simulink model "Lab1_open"  (R2024b)
settings: Solver=ode1  StartTime=0.0  StopTime=5  FixedStep=0.002  RelTol=1e-3  EnableMultiTasking=on
undefined symbols (not defined in the file or in its folder): HIL
libraries: quarc_library x3
settings Model: ExtModeTrigDuration=50001  Creator=Mounir  LastModifiedBy=dodso
settings SolverCC: AlgebraicLoopSolver=TrustRegion  PositivePriorityOrder=on
settings DataIOCC: LimitDataPoints=on  SaveFormat=Array  SaveOutput=off  SaveTime=off  ReturnWorkspaceOutputs=off
settings OptimizationCC: LifeSpan=inf
settings DebuggingCC: SolverPrmCheckMsg=warning  UnconnectedInputMsg=warning  UnconnectedOutputMsg=warning  UnconnectedLineMsg=warning  AllowSymbolicDim=off  SFUnexpectedBacktrackingDiag=warning  SFNoUnconditionalDefaultTransitionDiag=warning  SFExecutionAtInitializationDiag=none  ArithmeticOperatorsInVariantConditions=warning
settings HardwareCC: ProdBitPerPointer=32  ProdBitPerSizeT=32  ProdBitPerPtrDiffT=32  ProdLargestAtomicFloat=None  ProdIntDivRoundTo=Undefined  ProdEndianess=Unspecified  ProdWordSize=32  ProdHWDeviceType=32-bit Generic
settings ModelReferenceCC: EnableRefExpFcnMdlSchedulingChecks=on  PropagateSignalLabelsOutOfModel=off
settings SFSimCC: SimUseLocalCustomCode=off  CustomCodeUndefinedFunction=UseInterfaceOnly
settings RTWCC: Description=QUARC Win64 Target  SystemTargetFile=quarc_win64.tlc  TemplateMakefile=quarc_default_tmf  RTWUseLocalCustomCode=off  GPUComputeCapability=3.5
settings CodeAppCC: StateflowObjectComments=on
settings STFCustomTargetCC: TargetPreCompLibLocation=C:\PROGRA~3\QUARC\lib\2015b\win64\release  ConcurrentExecutionCompliant=on  CombineOutputUpdateFcns=on  SystemTargetFile=quarc_win64.tlc
settings GRTTargetCC: TargetPreCompLibLocation=C:\PROGRA~3\QUARC\lib\2015b\win64\release  TargetLangStandard=C89/C90 (ANSI)  ParMdlRefBuildCompliant=off  CompOptLevelCompliant=off  MatFileLogging=off  CPPClassGenCompliant=off  UseToolchainInfoCompliant=off  ExtMode=on  ExtModeMexFile=quarc_comm
settings ConfigComp: CovMetricSettings=dw  CovSaveCumulativeToWorkspaceVar=on  CovSaveSingleToWorkspaceVar=on  CovExternalEMLEnable=off  CovSFcnEnable=off

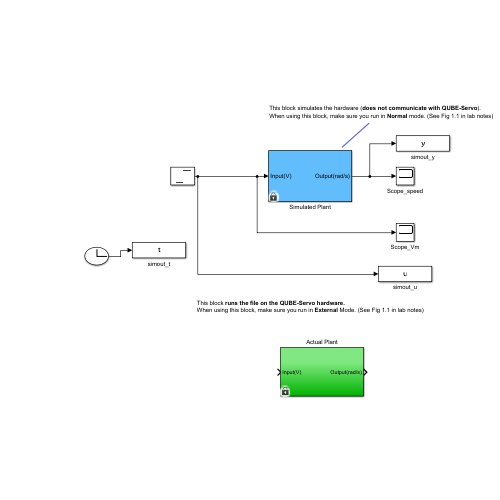
[thumbnail: Simulink's stored preview of the top-level diagram]
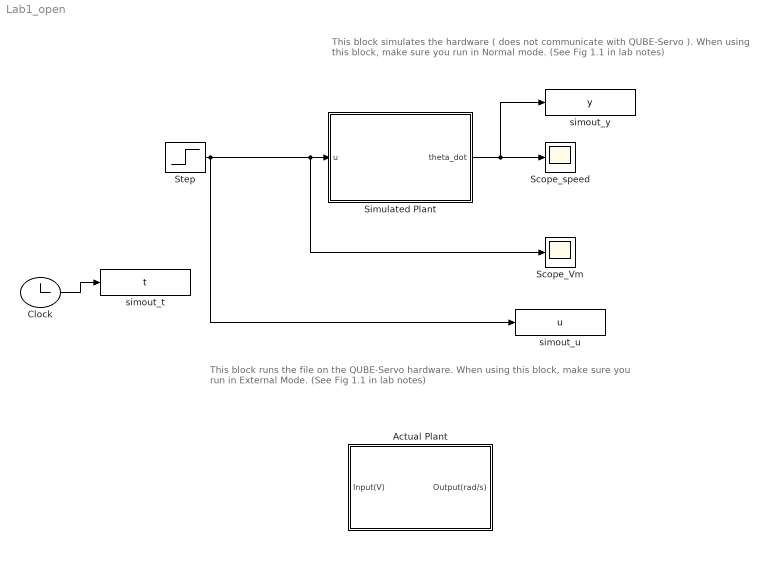
== system Lab1_open ==
  note: This block simulates the hardware ( does not communicate with QUBE-Servo ).
      | When using this block, make sure you run in Normal mode. (See Fig 1.1 in lab notes)
  note: This block runs the file on the QUBE-Servo hardware.
      | When using this block, make sure you run in External Mode. (See Fig 1.1 in lab notes)
  Actual Plant : Subsystem
  Clock : Clock
  Scope_Vm : Scope
  Scope_speed : Scope
  Simulated Plant : Subsystem
      mask Display:
      | %image('Qube.jpg')
      | port_label('input', 1, 'Input(V)')
      | port_label('output', 1, 'Output(rad/s)')
  Step : Step  After=2  SampleTime=0
  simout_t : ToWorkspace  VariableName=t  SampleTime=-1
  simout_u : ToWorkspace  VariableName=u  SampleTime=-1
  simout_y : ToWorkspace  VariableName=y  SampleTime=-1
  wires:
  Step/1 -> Simulated Plant/1(u), Scope_Vm/1, simout_u/1
  Simulated Plant/1(theta_dot) -> Scope_speed/1, simout_y/1
  Clock/1 -> simout_t/1

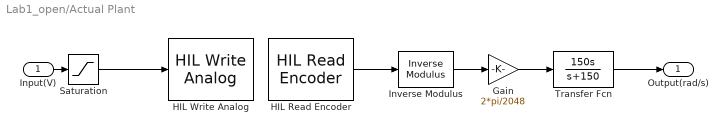
== system Lab1_open/Actual Plant ==
  Input(V) : Inport
  Gain : Gain  Gain=2*pi/2048
  HIL Read Encoder : quarc_library/Data Acquisition/Generic/Immediate I//O/HIL Read Encoder  object_name=HIL-1  channels=0  sample_time=qc_get_step_size  active=on  vector_output=off  data_type_mode=Inherit via back propagation  data_type=double
  HIL Write Analog : quarc_library/Data Acquisition/Generic/Immediate I//O/HIL Write Analog  object_name=HIL-1  channels=0  sample_time=-1  active=off  vector_input=off
  Inverse Modulus : quarc_library/Discontinuities/Inverse Modulus  modulus=65535  output_derivative=off  output_revolutions=off  max_x=Inf  min_x=-Inf
  Saturation : Saturate  UpperLimit=10  LowerLimit=-10
  Transfer Fcn : TransferFcn  Numerator=[150 0]  Denominator=[1 150]
  Output(rad/s) : Outport
  wires:
  HIL Read Encoder/1 -> Inverse Modulus/1
  Input(V)/1 -> Saturation/1
  Inverse Modulus/1 -> Gain/1
  Gain/1 -> Transfer Fcn/1
  Transfer Fcn/1 -> Output(rad/s)/1
  Saturation/1 -> HIL Write Analog/1

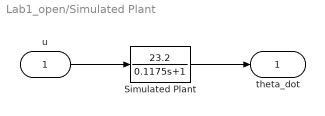
== system Lab1_open/Simulated Plant ==
  u : Inport
  Simulated Plant : TransferFcn  Numerator=[23.2]  Denominator=[0.1175 1]
  theta_dot : Outport
  wires:
  Simulated Plant/1 -> theta_dot/1
  u/1 -> Simulated Plant/1
